simulink model "prob_6"  (R2019b)
settings: Solver=VariableStepAuto  StartTime=0.0  StopTime=10.0  RelTol=1e-3
settings Model: Creator=kcalp  LastModifiedBy=kcalp

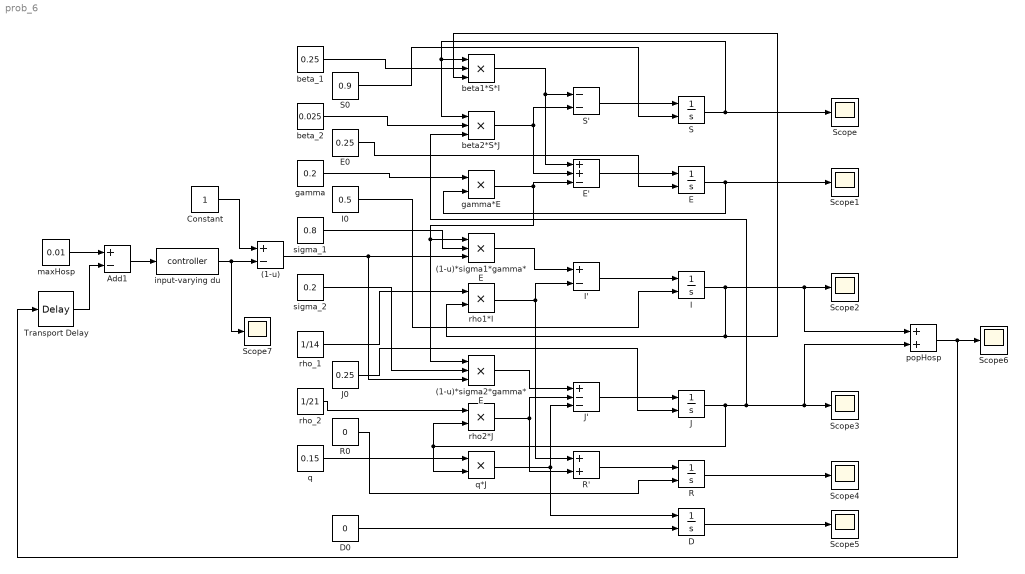
== system prob_6 ==
  (1-u) : Sum  Inputs=+-
  "(1-u)*sigma1*gamma*E " : Product  Inputs=3
  "(1-u)*sigma2*gamma*E " : Product  Inputs=3
  Add1 : Sum  Inputs=+-
  Constant : Constant
  D : Integrator  InitialConditionSource=external
  D0 : Constant  Value=0
  E : Integrator  InitialConditionSource=external
  "E' " : Sum  Inputs=++-
  "E0 " : Constant  Value=0.25
  "I " : Integrator  InitialConditionSource=external
  "I' " : Sum  Inputs=+-
  "I0 " : Constant  Value=0.5
  J : Integrator  InitialConditionSource=external
  "J' " : Sum  Inputs=+--
  "J0 " : Constant  Value=0.25
  R : Integrator  InitialConditionSource=external
  "R' " : Sum  Inputs=2
  R0 : Constant  Value=0
  S : Integrator  InitialConditionSource=external
  "S' " : Sum  Inputs=--
  "S0 " : Constant  Value=0.9
  Scope{,1..7} (8 alike) : Scope
  Transport Delay : TransportDelay
  "beta1*S*I " : Product  Inputs=3
  beta2*S*J : Product  Inputs=3
  "beta_1 " : Constant  Value=0.25
  "beta_2 " : Constant  Value=0.025
  "gamma " : Constant  Value=0.2
  "gamma*E " : Product
  input-varying du : MATLABFcn  MATLABFcn=controller
  "maxHosp " : Constant  Value=0.01
  popHosp : Sum
  q : Constant  Value=0.15
  q*J : Product
  rho1*I : Product
  rho2*J : Product
  rho_1 : Constant  Value=1/14
  "rho_2 " : Constant  Value=1/21
  sigma_1 : Constant  Value=0.8
  sigma_2 : Constant  Value=0.2
  wires:
  "I' "/1 -> "I "/1
  D0/1 -> D/2
  sigma_2/1 -> "(1-u)*sigma2*gamma*E "/2
  q*J/1 -> "J' "/3, D/1
  D/1 -> Scope5/1
  "I0 "/1 -> "I "/2
  rho1*I/1 -> "R' "/1, "I' "/2
  "J0 "/1 -> J/2
  J/1 -> beta2*S*J/3, Scope3/1, popHosp/2, rho2*J/2, q*J/2
  rho2*J/1 -> "J' "/2, "R' "/2
  rho_1/1 -> rho1*I/1
  q/1 -> q*J/1
  E/1 -> Scope1/1, "gamma*E "/2
  "(1-u)*sigma2*gamma*E "/1 -> "J' "/1
  R/1 -> Scope4/1
  R0/1 -> R/2
  "beta_1 "/1 -> "beta1*S*I "/2
  "J' "/1 -> J/1
  "(1-u)*sigma1*gamma*E "/1 -> "I' "/1
  "gamma*E "/1 -> "(1-u)*sigma1*gamma*E "/1, "(1-u)*sigma2*gamma*E "/1, "E' "/3
  "I "/1 -> "beta1*S*I "/3, rho1*I/2, Scope2/1, popHosp/1
  "R' "/1 -> R/1
  "E0 "/1 -> E/2
  "beta1*S*I "/1 -> "E' "/1, "S' "/1
  sigma_1/1 -> "(1-u)*sigma1*gamma*E "/2
  "rho_2 "/1 -> rho2*J/1
  beta2*S*J/1 -> "S' "/2, "E' "/2
  "S0 "/1 -> S/2
  "beta_2 "/1 -> beta2*S*J/2
  S/1 -> Scope/1, "beta1*S*I "/1, beta2*S*J/1
  "S' "/1 -> S/1
  "gamma "/1 -> "gamma*E "/1
  "E' "/1 -> E/1
  (1-u)/1 -> "(1-u)*sigma2*gamma*E "/3, "(1-u)*sigma1*gamma*E "/3
  Constant/1 -> (1-u)/1
  input-varying du/1 -> Scope7/1, (1-u)/2
  Add1/1 -> input-varying du/1
  popHosp/1 -> Scope6/1, Transport Delay/1
  "maxHosp "/1 -> Add1/1
  Transport Delay/1 -> Add1/2
